simulink model "EMR"  (R2022b)
settings: Solver=ode45  StartTime=0.0  StopTime=1220  MaxStep=1  RelTol=1e-3  EnableMultiTasking=on
values from neighbouring files (symbols this model uses):
  alpha = linspace(0,2*pi)    [control_plot.m]
  Ld = 0.12e-3    (= 0.00012)    [control_plot.m]
  Lq = 0.24e-3    (= 0.00024)    [control_plot.m]
  Rs = 0.135    [control_plot.m]
undefined symbols (not defined in the file or in its folder): A, Af, B, Cd, fr, g, K, Ki_id, Ki_iq, Ki_v, Kp_id, Kp_iq, Kp_v, kred, lambdam, mv, Npar, Nser, p, Q, rho, Rint, rw, vair
libraries: simulink x4
settings Model: Creator=Daniel Montesinos  LastModifiedBy=danie
settings SolverCC: AlgebraicLoopSolver=TrustRegion
settings DataIOCC: LimitDataPoints=on  SaveFormat=Array  SignalLoggingSaveFormat=ModelDataLogs  ReturnWorkspaceOutputs=off
settings OptimizationCC: ExpressionDepthLimit=2147483647  LifeSpan=inf
settings DebuggingCC: UnderspecifiedInitializationDetection=Classic  MergeDetectMultiDrivingBlocksExec=none  SolverPrmCheckMsg=warning  FcnCallInpInsideContextMsg=warning  UnconnectedInputMsg=warning  UnconnectedOutputMsg=warning  UnconnectedLineMsg=warning  AllowSymbolicDim=off  StateNameClashWarn=warning  SFUnexpectedBacktrackingDiag=warning  SFNoUnconditionalDefaultTransitionDiag=warning  SFExecutionAtInitializationDiag=none  SFMachineParentedDataDiag=warning  ArithmeticOperatorsInVariantConditions=warning
settings HardwareCC: ProdBitPerPointer=32  ProdBitPerSizeT=32  ProdBitPerPtrDiffT=32  ProdLargestAtomicFloat=None  ProdIntDivRoundTo=Undefined  ProdEndianess=Unspecified  ProdWordSize=32  ProdHWDeviceType=32-bit Generic
settings ModelReferenceCC: EnableRefExpFcnMdlSchedulingChecks=on  PropagateSignalLabelsOutOfModel=off
settings SFSimCC: SimUseLocalCustomCode=off  CustomCodeUndefinedFunction=UseInterfaceOnly
settings RTWCC: RTWUseLocalCustomCode=off  DLArmComputeVersion=19.05
settings CodeAppCC: StateflowObjectComments=on
settings GRTTargetCC: TargetLangStandard=C89/C90 (ANSI)  CombineOutputUpdateFcns=off  GRTInterface=on
settings ConfigComp: CovMetricSettings=dw  CovSaveCumulativeToWorkspaceVar=on  CovSaveSingleToWorkspaceVar=on  CovExternalEMLEnable=off  CovSFcnEnable=off

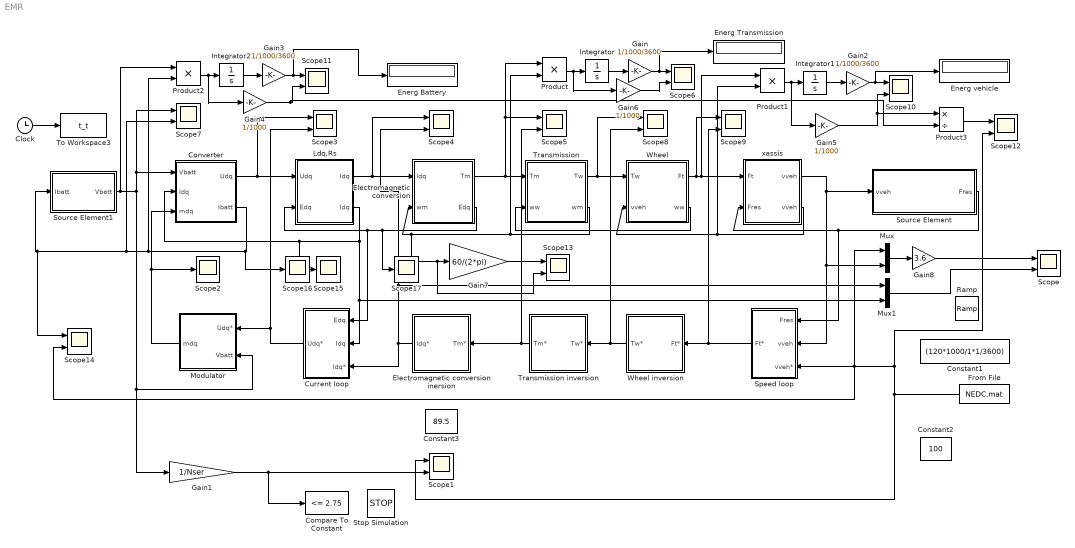
== system EMR ==
  Clock : Clock
  Compare To Constant : simulink/Logic and Bit Operations/Compare To Constant  relop=<=  const=2.75  OutDataTypeStr=boolean
  Constant1 : Constant  Value=(120*1000/1*1/3600)
  Constant2 : Constant  Value=100
  Constant3 : Constant  Value=89.5
  Converter : Subsystem  AncestorBlock=simulink/REM/EC Elec  mask(Hacheur){}
      settings: LibrarySourceBlock=simulink/REM/EC Elec
      mask Display: plot(0,0,100,100,[10,10,90,90,10],[90,10,10,90,90])
  Current loop : Subsystem  AncestorBlock=simulink/SMC/Asservissement Correcteur IP
      settings: LibrarySourceBlock=|
      | simulink/SMC/Asservissement
      | Correcteur IP
      mask Display: plot(0,0,100,100, [10,30,90,70,10,90],[90,10,10,90,90,10])
  Electromagnetic conversion : Subsystem  AncestorBlock=simulink/REM/EC EM
      settings: LibrarySourceBlock=simulink/REM/EC EM
      mask Display: plot(0,0,100,100, 1.4*[50,57.68,60.77,63.08,64.97,66.58,68,69.26,70.4, 	71.42,72.36,78.28,80,78.28,72.36,71.42,70.4, 	69.26,68,66.58,64.97,63.08,60.77,57.68,50,42.32, 	39.23,36.92,35.03,33.42,32,30.74,29.6,28.58, 	27.64,21.72,20,21.72,27.64,28.58,29.6,30.74,32, 	33.42,35.03,36.92,39.23,42.32,50]-20, 1.4*[20,21,22,23,24,25,26,27,28,29,30,40,50,60,70,71,72, 	73,74,75,76,77,78,79,80,79,78,77,76,75,74,73,72, 	71,70,60,50,40,30,29,28,27,26,25,24,23,22,21,20]-20)
  Electromagnetic conversion inersion : Subsystem  AncestorBlock=simulink/SMC/Inversion EC avec mesure
      settings: LibrarySourceBlock=|
      | simulink/SMC/Inversion EC
      | avec mesure
      mask Display: plot(0,0,100,100,[10,30,90,70,10],[90,10,10,90,90])
  Energ Battery : Display
  Energ Transmission : Display
  Energ vehicle : Display
  From File : FromFile  FileName=NEDC.mat  SampleTime=0
  Gain : Gain  Gain=1/1000/3600
  Gain1 : Gain  Gain=1/Nser
  Gain2 : Gain  Gain=1/1000/3600
  Gain3 : Gain  Gain=1/1000/3600
  Gain4 : Gain  Gain=1/1000
  Gain5 : Gain  Gain=1/1000
  Gain6 : Gain  Gain=1/1000
  Gain7 : Gain  Gain=60/(2*pi)
  Gain8 : Gain  Gain=3.6
  Integrator : Integrator
  Integrator1 : Integrator
  Integrator2 : Integrator
  Ldq,Rs : Subsystem  AncestorBlock=simulink/REM/EA  mask(CM){}
      settings: LibrarySourceBlock=simulink/REM/EA
      mask Display: plot(0,0,100,100,[10,10,90,90,10],[90,10,10,90,90], [10,90],[10,90])
  Modulator : Subsystem  AncestorBlock=simulink/SMC/Inversion EC avec mesure
      settings: LibrarySourceBlock=|
      | simulink/SMC/Inversion EC
      | avec mesure
      mask Display: plot(0,0,100,100,[10,30,90,70,10],[90,10,10,90,90])
  Mux : Mux  Inputs=2
  Mux1 : Mux  Inputs=2
  Product : Product
  Product1 : Product
  Product2 : Product
  Product3 : Product  Inputs=*/
  Ramp : simulink/Sources/Ramp  slope=100/3.6/10  start=0  InitialOutput=0
  Scope{,1,3..14} (14 alike) : Scope  NumInputPorts=2
  Scope{2,15..17} (4 alike) : Scope
  Source Element : Subsystem  AncestorBlock=simulink/REM/SE
      settings: LibrarySourceBlock=simulink/REM/SE
      mask Display:
      | plot(0,0,100,100, 1.2*[50,57.68,60.77,63.08,64.97,66.58,68,69.26,70.4, 	71.42,72.36,78.28,80,78.28,72.36,71.42,70.4, 	69.26,68,66.58,64.97,63.08,60.77,57.68,50,42.32, 	39.23,36.92,35.03,33.42,32,30.74,29.6,28.58, 	27.64,21.72,20,21.72,27.64,28.58,29.6,30.74,32, 	33.42,35.03,36.92,39.23,42.32,50]-10, 1.2*[20,21,22,23,24,25,26,27,28,29,30,40,50,60,70,71,72, 	73,74,75,76,77,78,79,80,79,78,77,76,75,74,73,72, 	71,70,60,50,40,30,29,28,27,26,25,24,23,22,21,20]-10)
      | disp('Source')
  Source Element1 : Subsystem  AncestorBlock=simulink/REM/SE
      settings: LibrarySourceBlock=simulink/REM/SE
      mask Display:
      | plot(0,0,100,100, 1.2*[50,57.68,60.77,63.08,64.97,66.58,68,69.26,70.4, 	71.42,72.36,78.28,80,78.28,72.36,71.42,70.4, 	69.26,68,66.58,64.97,63.08,60.77,57.68,50,42.32, 	39.23,36.92,35.03,33.42,32,30.74,29.6,28.58, 	27.64,21.72,20,21.72,27.64,28.58,29.6,30.74,32, 	33.42,35.03,36.92,39.23,42.32,50]-10, 1.2*[20,21,22,23,24,25,26,27,28,29,30,40,50,60,70,71,72, 	73,74,75,76,77,78,79,80,79,78,77,76,75,74,73,72, 	71,70,60,50,40,30,29,28,27,26,25,24,23,22,21,20]-10)
      | disp('Source')
  Speed loop : Subsystem  AncestorBlock=simulink/SMC/Asservissement Correcteur IP
      settings: LibrarySourceBlock=|
      | simulink/SMC/Asservissement
      | Correcteur IP
      mask Display: plot(0,0,100,100, [10,30,90,70,10,90],[90,10,10,90,90,10])
  Stop Simulation : Stop
  To Workspace3 : ToWorkspace  VariableName=t_t  SampleTime=-1
  Transmission : Subsystem  AncestorBlock=simulink/REM/EC Elec  mask(Hacheur){}
      settings: LibrarySourceBlock=simulink/REM/EC Elec
      mask Display: plot(0,0,100,100,[10,10,90,90,10],[90,10,10,90,90])
  Transmission inversion : Subsystem  AncestorBlock=simulink/SMC/Inversion EC avec mesure
      settings: LibrarySourceBlock=|
      | simulink/SMC/Inversion EC
      | avec mesure
      mask Display: plot(0,0,100,100,[10,30,90,70,10],[90,10,10,90,90])
  Wheel : Subsystem  AncestorBlock=simulink/REM/EC Elec  mask(Hacheur){}
      settings: LibrarySourceBlock=simulink/REM/EC Elec
      mask Display: plot(0,0,100,100,[10,10,90,90,10],[90,10,10,90,90])
  Wheel inversion : Subsystem  AncestorBlock=simulink/SMC/Inversion EC avec mesure
      settings: LibrarySourceBlock=|
      | simulink/SMC/Inversion EC
      | avec mesure
      mask Display: plot(0,0,100,100,[10,30,90,70,10],[90,10,10,90,90])
  xassís : Subsystem  AncestorBlock=simulink/REM/EA  mask(CM){}
      settings: LibrarySourceBlock=simulink/REM/EA
      mask Display: plot(0,0,100,100,[10,10,90,90,10],[90,10,10,90,90], [10,90],[10,90])
  wires:
  Clock/1 -> To Workspace3/1
  From File/1 -> Scope12/2, Scope14/2, Speed loop/3(vveh*), Mux/1, Scope1/1
  xassís/1(vveh) -> Speed loop/2(vveh), Mux/2, Source Element/1(vveh)
  Source Element/1(Fres) -> xassís/2(Fres), Speed loop/1(Fres)
  Mux/1 -> Gain8/1
  xassís/2("vveh ") -> Product1/2, Wheel/2(vveh)
  Transmission/1(Tw) -> Scope8/1, Wheel/1(Tw)
  Wheel/2(ww) -> Transmission/2(ww)
  Wheel inversion/1(Tw*) -> Scope8/2, Transmission inversion/1(Tw*)
  Transmission/2(wm) -> Scope13/2, Gain7/1, Electromagnetic conversion/2(wm), Product/2
  Electromagnetic conversion/1(Tm) -> Product/1, Scope5/1, Transmission/1(Tm)
  Electromagnetic conversion/2(Edq) -> Scope17/1, Ldq,Rs/2(Edq), Current loop/1(Edq)
  Electromagnetic conversion inersion/1(Idq*) -> Current loop/3(Idq*), Scope4/2, Mux1/1
  Transmission inversion/1(Tm*) -> Electromagnetic conversion inersion/1(Tm*), Scope5/2
  Modulator/1(mdq) -> Scope2/1, Converter/3(mdq)
  Converter/2(Ibatt) -> Scope16/1, Product2/2, Scope7/2, Scope14/1, Source Element1/1(Ibatt)
  Source Element1/1(Vbatt) -> Product2/1, Gain1/1, Modulator/2(Vbatt), Scope7/1, Converter/1(Vbatt)
  Speed loop/1(Ft*) -> Scope9/2, Wheel inversion/1(Ft*)
  Wheel/1(Ft) -> Scope9/1, Product1/1, xassís/1(Ft)
  Product/1 -> Gain6/1, Integrator/1
  Current loop/1(Udq*) -> Scope3/2, Modulator/1(Udq*)
  Converter/1(Udq) -> Scope3/1, Ldq,Rs/1(Udq)
  Integrator/1 -> Gain/1
  Gain/1 -> Energ Transmission/1, Scope6/1
  Gain1/1 -> Compare To Constant/1, Scope1/2
  Product1/1 -> Gain5/1, Integrator1/1
  Gain2/1 -> Energ vehicle/1, Scope10/1
  Integrator1/1 -> Gain2/1
  Product2/1 -> Gain4/1, Integrator2/1
  Gain3/1 -> Energ Battery/1, Scope11/1
  Integrator2/1 -> Gain3/1
  Gain4/1 -> Product3/2, Scope11/2
  Gain5/1 -> Product3/1, Scope10/2
  Product3/1 -> Scope12/1
  Gain6/1 -> Scope6/2
  Ldq,Rs/1("Idq ") -> Scope4/1, Electromagnetic conversion/1(Idq)
  Ldq,Rs/2(Idq) -> Mux1/2, Current loop/2(Idq), Scope15/1, Converter/2(Idq)
  Gain7/1 -> Scope13/1
  Gain8/1 -> Scope/1
  Mux1/1 -> Scope/2

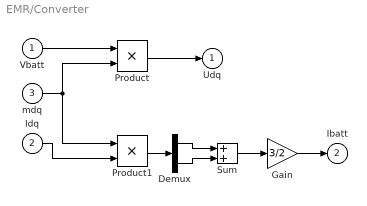
== system EMR/Converter ==
  Vbatt : Inport
  Idq : Inport  Port=2
  mdq : Inport  Port=3
  Demux : Demux  Outputs=2
  Gain : Gain  Gain=3/2
  Product : Product
  Product1 : Product
  Sum : Sum
  Udq : Outport  InitialOutput=0  VectorParamsAs1DForOutWhenUnconnected=off
  Ibatt : Outport  Port=2  InitialOutput=0  VectorParamsAs1DForOutWhenUnconnected=off
  wires:
  Vbatt/1 -> Product/1
  mdq/1 -> Product1/1, Product/2
  Product/1 -> Udq/1
  Product1/1 -> Demux/1
  Demux/1 -> Sum/1
  Demux/2 -> Sum/2
  Sum/1 -> Gain/1
  Gain/1 -> Ibatt/1
  Idq/1 -> Product1/2

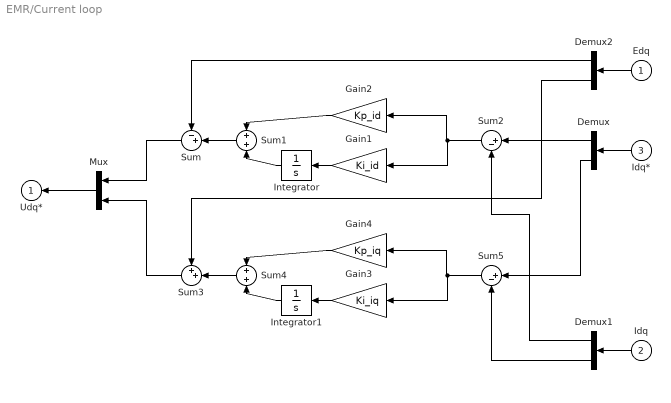
== system EMR/Current loop ==
  Edq : Inport
  Idq : Inport  Port=2
  Idq* : Inport  Port=3
  Demux : Demux  Outputs=2
  Demux1 : Demux  Outputs=2
  Demux2 : Demux  Outputs=2
  Gain1 : Gain  Gain=Ki_id
  Gain2 : Gain  Gain=Kp_id
  Gain3 : Gain  Gain=Ki_iq
  Gain4 : Gain  Gain=Kp_iq
  Integrator : Integrator
  Integrator1 : Integrator
  Mux : Mux  Inputs=2
  Sum : Sum  Inputs=-+|
  Sum1 : Sum
  Sum2 : Sum  Inputs=|+-
  Sum3 : Sum  Inputs=++|
  Sum4 : Sum
  Sum5 : Sum  Inputs=|+-
  Udq* : Outport  InitialOutput=0  VectorParamsAs1DForOutWhenUnconnected=off
  wires:
  Sum1/1 -> Sum/2
  Gain2/1 -> Sum1/1
  Integrator/1 -> Sum1/2
  Gain1/1 -> Integrator/1
  Sum2/1 -> Gain1/1, Gain2/1
  Integrator1/1 -> Sum4/2
  Gain3/1 -> Integrator1/1
  Gain4/1 -> Sum4/1
  Sum5/1 -> Gain3/1, Gain4/1
  Sum4/1 -> Sum3/2
  Idq*/1 -> Demux/1
  Demux/1 -> Sum2/1
  Demux/2 -> Sum5/1
  Idq/1 -> Demux1/1
  Demux1/1 -> Sum2/2
  Demux1/2 -> Sum5/2
  Edq/1 -> Demux2/1
  Demux2/2 -> Sum3/1
  Sum/1 -> Mux/1
  Sum3/1 -> Mux/2
  Mux/1 -> Udq*/1
  Demux2/1 -> Sum/1

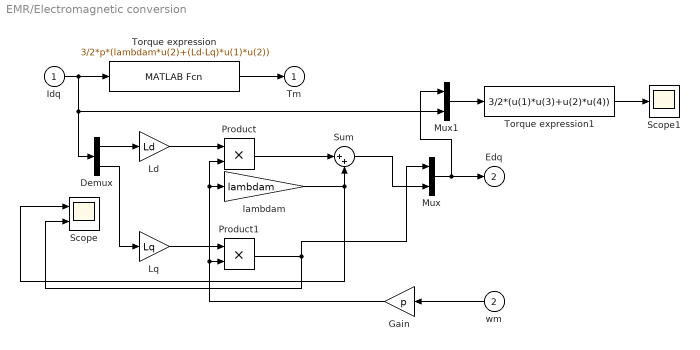
== system EMR/Electromagnetic conversion ==
  Idq : Inport
  wm : Inport  Port=2
  Demux : Demux  Outputs=2
  Gain : Gain  Gain=p
  Ld : Gain  Gain=Ld
  Lq : Gain  Gain=Lq
  Mux : Mux  Inputs=2
  Mux1 : Mux  Inputs=2
  Product : Product
  Product1 : Product
  Scope : Scope  NumInputPorts=2
  Scope1 : Scope
  Sum : Sum  Inputs=|++
  Torque expression : MATLABFcn  MATLABFcn=3/2*p*(lambdam*u(2)+(Ld-Lq)*u(1)*u(2))
  Torque expression1 : MATLABFcn  MATLABFcn=3/2*(u(1)*u(3)+u(2)*u(4))
  lambdam : Gain  Gain=lambdam
  Tm : Outport  InitialOutput=0  VectorParamsAs1DForOutWhenUnconnected=off
  Edq : Outport  Port=2  InitialOutput=0  VectorParamsAs1DForOutWhenUnconnected=off
  wires:
  Torque expression/1 -> Tm/1
  Idq/1 -> Mux1/2, Demux/1, Torque expression/1
  Demux/1 -> Ld/1
  Demux/2 -> Lq/1
  Ld/1 -> Product/1
  wm/1 -> Gain/1
  Lq/1 -> Product1/1
  Product/1 -> Sum/1
  lambdam/1 -> Scope/1, Sum/2
  Product1/1 -> Scope/2, Mux/1
  Mux/1 -> Mux1/1, Edq/1
  Mux1/1 -> Torque expression1/1
  Torque expression1/1 -> Scope1/1
  Sum/1 -> Mux/2
  Gain/1 -> Product/2, lambdam/1, Product1/2

== system EMR/Electromagnetic conversion inersion ==
  Tm* : Inport
  Constant : Constant  Value=0
  Gain1 : Gain  Gain=2/(3*p*lambdam)
  Mux : Mux  Inputs=2
  Idq* : Outport  InitialOutput=0  VectorParamsAs1DForOutWhenUnconnected=off
  wires:
  Tm*/1 -> Gain1/1
  Gain1/1 -> Mux/2
  Mux/1 -> Idq*/1
  Constant/1 -> Mux/1

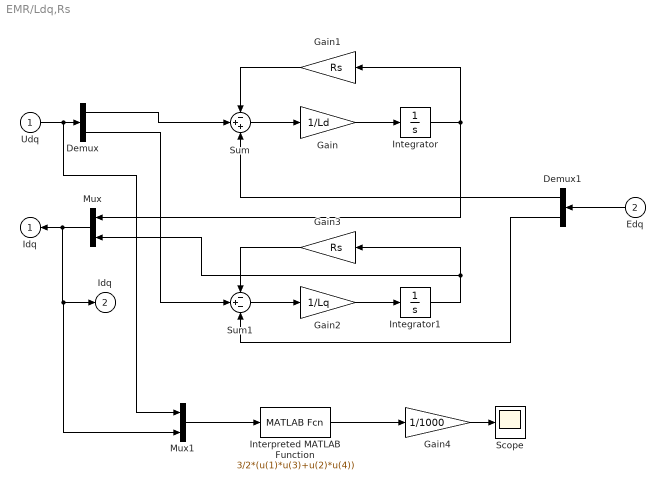
== system EMR/Ldq,Rs ==
  Udq : Inport
  Edq : Inport  Port=2
  Demux : Demux  Outputs=2
  Demux1 : Demux  Outputs=2
  Gain : Gain  Gain=1/Ld
  Gain1 : Gain  Gain=Rs
  Gain2 : Gain  Gain=1/Lq
  Gain3 : Gain  Gain=Rs
  Gain4 : Gain  Gain=1/1000
  Integrator : Integrator
  Integrator1 : Integrator
  Interpreted MATLAB Function : MATLABFcn  MATLABFcn=3/2*(u(1)*u(3)+u(2)*u(4))
  Mux : Mux  Inputs=2
  Mux1 : Mux  Inputs=2
  Scope : Scope
  Sum : Sum  Inputs=-++
  Sum1 : Sum  Inputs=-+-
  "Idq " : Outport  InitialOutput=0  VectorParamsAs1DForOutWhenUnconnected=off
  Idq : Outport  Port=2  InitialOutput=0  VectorParamsAs1DForOutWhenUnconnected=off
  wires:
  Integrator/1 -> Mux/1, Gain1/1
  Gain/1 -> Integrator/1
  Sum/1 -> Gain/1
  Gain1/1 -> Sum/1
  Gain3/1 -> Sum1/1
  Gain2/1 -> Integrator1/1
  Integrator1/1 -> Gain3/1, Mux/2
  Sum1/1 -> Gain2/1
  Udq/1 -> Mux1/1, Demux/1
  Demux/1 -> Sum/2
  Demux/2 -> Sum1/2
  Mux/1 -> Mux1/2, Idq/1, "Idq "/1
  Edq/1 -> Demux1/1
  Mux1/1 -> Interpreted MATLAB Function/1
  Interpreted MATLAB Function/1 -> Gain4/1
  Gain4/1 -> Scope/1
  Demux1/1 -> Sum/3
  Demux1/2 -> Sum1/3

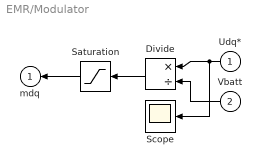
== system EMR/Modulator ==
  Udq* : Inport
  Vbatt : Inport  Port=2
  Divide : Product  Inputs=*/
  Saturation : Saturate  UpperLimit=1  LowerLimit=-1
  Scope : Scope
  mdq : Outport  InitialOutput=0  VectorParamsAs1DForOutWhenUnconnected=off
  wires:
  Divide/1 -> Saturation/1
  Udq*/1 -> Scope/1, Divide/1
  Vbatt/1 -> Divide/2
  Saturation/1 -> mdq/1

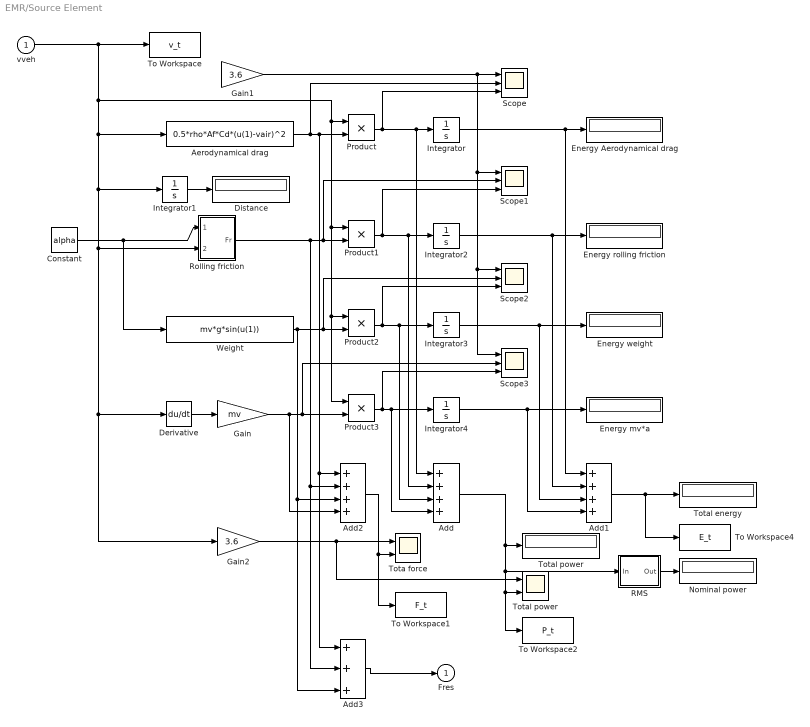
== system EMR/Source Element ==
  vveh : Inport
  Add : Sum  Inputs=++++
  Add1 : Sum  Inputs=++++
  Add2 : Sum  Inputs=++++
  Add3 : Sum  Inputs=+++
  Aerodynamical drag : Fcn  Expr=0.5*rho*Af*Cd*(u(1)-vair)^2
  Constant : Constant  Value=alpha
  Derivative : Derivative
  Distance : Display
  Energy Aerodynamical drag : Display
  Energy mv*a : Display
  Energy rolling friction : Display
  Energy weight : Display
  Gain : Gain  Gain=mv
  Gain1 : Gain  Gain=3.6
  Gain2 : Gain  Gain=3.6
  Integrator{,1..4} (5 alike) : Integrator
  Nominal power : Display
  Product{,1..3} (4 alike) : Product  RndMeth=Zero
  RMS : Subsystem
  Rolling friction : Subsystem
  Scope{,1..3} (4 alike) : Scope  NumInputPorts=3
  To Workspace : ToWorkspace  VariableName=v_t  SampleTime=-1
  To Workspace1 : ToWorkspace  VariableName=F_t  SampleTime=-1
  To Workspace2 : ToWorkspace  VariableName=P_t  SampleTime=-1
  To Workspace4 : ToWorkspace  VariableName=E_t  SampleTime=-1
  Tota force : Scope  NumInputPorts=2
  Total energy : Display
  Total power : Scope  NumInputPorts=2
  "Total power " : Display
  Weight : Fcn  Expr=mv*g*sin(u(1))
  Fres : Outport  InitialOutput=0  VectorParamsAs1DForOutWhenUnconnected=off
  wires:
  Aerodynamical drag/1 -> Scope/2, Product/2, Add2/1, Add3/1
  Product/1 -> Scope/3, Integrator/1, Add/1
  Integrator1/1 -> Distance/1
  Constant/1 -> Weight/1, Rolling friction/1(alpha)
  Product1/1 -> Scope1/3, Integrator2/1, Add/2
  Product2/1 -> Scope2/3, Integrator3/1, Add/3
  Weight/1 -> Product2/2, Scope2/2, Add2/3, Add3/3
  Integrator/1 -> Energy Aerodynamical drag/1, Add1/1
  Integrator3/1 -> Energy weight/1, Add1/3
  Integrator2/1 -> Energy rolling friction/1, Add1/2
  Gain/1 -> Product3/2, Scope3/2, Add2/4
  Product3/1 -> Scope3/3, Integrator4/1, Add/4
  Integrator4/1 -> Energy mv*a/1, Add1/4
  Add/1 -> "Total power "/1, Total power/2, To Workspace2/1, RMS/1(In)
  Add1/1 -> Total energy/1, To Workspace4/1
  Add2/1 -> Tota force/2, To Workspace1/1
  Rolling friction/1(Fr) -> Product1/2, Scope1/2, Add2/2, Add3/2
  Gain1/1 -> Scope3/1, Scope2/1, Scope1/1, Scope/1
  Gain2/1 -> Total power/1, Tota force/1
  RMS/1(Out) -> Nominal power/1
  Derivative/1 -> Gain/1
  vveh/1 -> To Workspace/1, Aerodynamical drag/1, Integrator1/1, Derivative/1, Gain2/1, Rolling friction/2(vveh), Product/1, Product1/1, Product2/1, Product3/1
  Add3/1 -> Fres/1

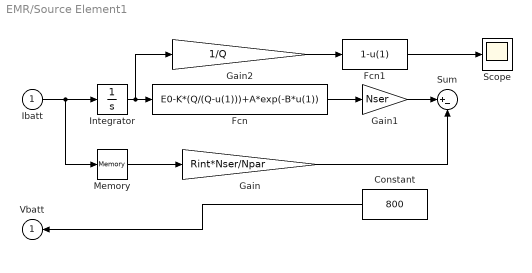
== system EMR/Source Element1 ==
  Ibatt : Inport
  Constant : Constant  Value=800
  Fcn : Fcn  Expr=E0-K*(Q/(Q-u(1)))+A*exp(-B*u(1))
  Fcn1 : Fcn  Expr=1-u(1)
  Gain : Gain  Gain=Rint*Nser/Npar
  Gain1 : Gain  Gain=Nser
  Gain2 : Gain  Gain=1/Q
  Integrator : Integrator
  Memory : Memory
  Scope : Scope
  Sum : Sum  Inputs=|+-
  Vbatt : Outport  InitialOutput=0  VectorParamsAs1DForOutWhenUnconnected=off
  wires:
  Integrator/1 -> Gain2/1, Fcn/1
  Gain/1 -> Sum/2
  Ibatt/1 -> Memory/1, Integrator/1
  Fcn/1 -> Gain1/1
  Gain1/1 -> Sum/1
  Memory/1 -> Gain/1
  Gain2/1 -> Fcn1/1
  Fcn1/1 -> Scope/1
  Constant/1 -> Vbatt/1

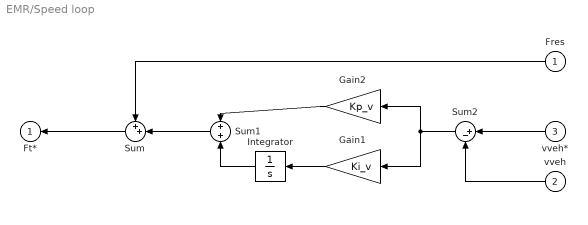
== system EMR/Speed loop ==
  Fres : Inport
  vveh : Inport  Port=2
  vveh* : Inport  Port=3
  Gain1 : Gain  Gain=Ki_v
  Gain2 : Gain  Gain=Kp_v
  Integrator : Integrator
  Sum : Sum  Inputs=++|
  Sum1 : Sum
  Sum2 : Sum  Inputs=|+-
  Ft* : Outport  InitialOutput=0  VectorParamsAs1DForOutWhenUnconnected=off
  wires:
  Sum/1 -> Ft*/1
  Fres/1 -> Sum/1
  Gain1/1 -> Integrator/1
  Integrator/1 -> Sum1/2
  Gain2/1 -> Sum1/1
  Sum1/1 -> Sum/2
  Sum2/1 -> Gain2/1, Gain1/1
  vveh*/1 -> Sum2/1
  vveh/1 -> Sum2/2

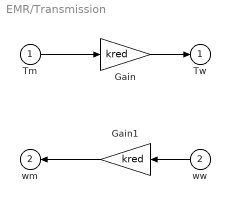
== system EMR/Transmission ==
  Tm : Inport
  ww : Inport  Port=2
  Gain : Gain  Gain=kred
  Gain1 : Gain  Gain=kred
  Tw : Outport  InitialOutput=0  VectorParamsAs1DForOutWhenUnconnected=off
  wm : Outport  Port=2  InitialOutput=0  VectorParamsAs1DForOutWhenUnconnected=off
  wires:
  Tm/1 -> Gain/1
  Gain/1 -> Tw/1
  Gain1/1 -> wm/1
  ww/1 -> Gain1/1

== system EMR/Transmission inversion ==
  Tw* : Inport
  Gain : Gain  Gain=1/kred
  Tm* : Outport  InitialOutput=0  VectorParamsAs1DForOutWhenUnconnected=off
  wires:
  Tw*/1 -> Gain/1
  Gain/1 -> Tm*/1

== system EMR/Wheel ==
  Tw : Inport
  vveh : Inport  Port=2
  Gain : Gain  Gain=1/rw
  Gain1 : Gain  Gain=1/rw
  Ft : Outport  InitialOutput=0  VectorParamsAs1DForOutWhenUnconnected=off
  ww : Outport  Port=2  InitialOutput=0  VectorParamsAs1DForOutWhenUnconnected=off
  wires:
  Tw/1 -> Gain/1
  Gain/1 -> Ft/1
  Gain1/1 -> ww/1
  vveh/1 -> Gain1/1

== system EMR/Wheel inversion ==
  Ft* : Inport
  Gain : Gain  Gain=rw
  Tw* : Outport  InitialOutput=0  VectorParamsAs1DForOutWhenUnconnected=off
  wires:
  Gain/1 -> Tw*/1
  Ft*/1 -> Gain/1

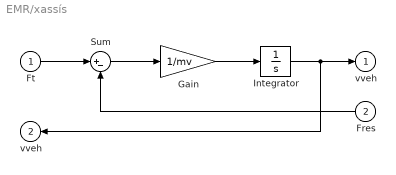
== system EMR/xassís ==
  Ft : Inport
  Fres : Inport  Port=2
  Gain : Gain  Gain=1/mv
  Integrator : Integrator
  Sum : Sum  Inputs=|+-
  vveh : Outport  InitialOutput=0  VectorParamsAs1DForOutWhenUnconnected=off
  "vveh " : Outport  Port=2  InitialOutput=0  VectorParamsAs1DForOutWhenUnconnected=off
  wires:
  Ft/1 -> Sum/1
  Fres/1 -> Sum/2
  Sum/1 -> Gain/1
  Gain/1 -> Integrator/1
  Integrator/1 -> vveh/1, "vveh "/1

== system EMR/Source Element/RMS ==
  In : Inport
  Gain3 : Gain  Gain=1/1220
  Integrator5 : Integrator
  Product4 : Product  RndMeth=Zero
  Sqrt : Sqrt
  Out : Outport  VectorParamsAs1DForOutWhenUnconnected=off
  wires:
  Product4/1 -> Integrator5/1
  Integrator5/1 -> Gain3/1
  Gain3/1 -> Sqrt/1
  In/1 -> Product4/2, Product4/1
  Sqrt/1 -> Out/1

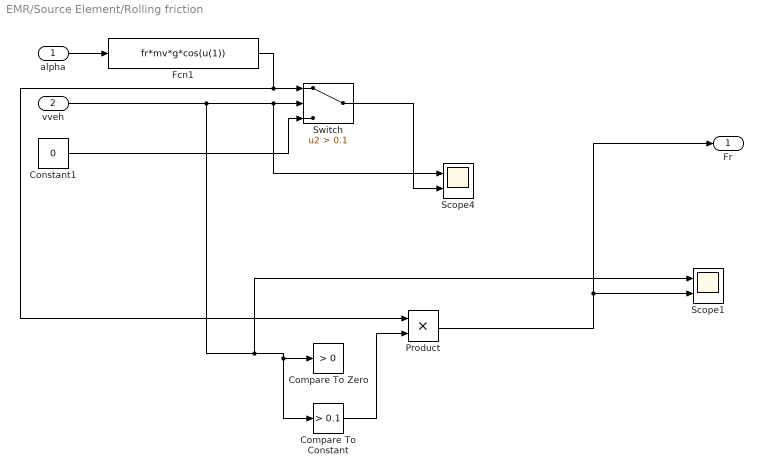
== system EMR/Source Element/Rolling friction ==
  alpha : Inport
  vveh : Inport  Port=2
  Compare To Constant : simulink/Logic and Bit Operations/Compare To Constant  relop=>  const=0.1  OutDataTypeStr=boolean
  Compare To Zero : simulink/Logic and Bit Operations/Compare To Zero  relop=>  OutDataTypeStr=boolean  ZeroCross=off
  Constant1 : Constant  Value=0
  Fcn1 : Fcn  Expr=fr*mv*g*cos(u(1))
  Product : Product
  Scope1 : Scope  NumInputPorts=2
  Scope4 : Scope  NumInputPorts=2
  Switch : Switch  Criteria=u2 > Threshold  Threshold=0.1  SaturateOnIntegerOverflow=off  InputSameDT=off
  Fr : Outport  VectorParamsAs1DForOutWhenUnconnected=off
  wires:
  alpha/1 -> Fcn1/1
  Switch/1 -> Scope4/2
  vveh/1 -> Scope1/1, Compare To Constant/1, Compare To Zero/1, Switch/2, Scope4/1
  Fcn1/1 -> Switch/1, Product/1
  Constant1/1 -> Switch/3
  Compare To Constant/1 -> Product/2
  Product/1 -> Scope1/2, Fr/1
